simulink model "balanceCar3"  (R2023b)
settings: Solver=VariableStepAuto  StartTime=0.0  StopTime=20  RelTol=1e-3
settings Model: SimulationMode=accelerator  Creator=xjtu  LastModifiedBy=xjtu

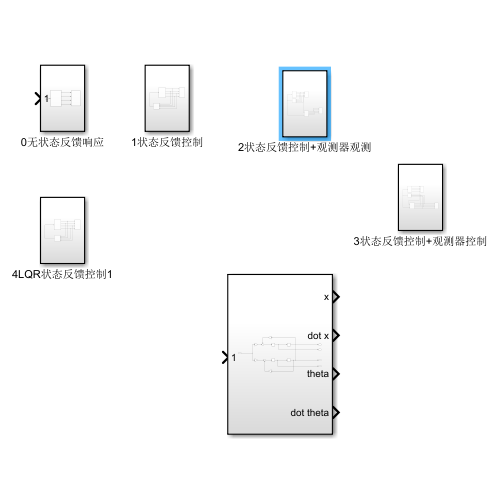
[thumbnail: Simulink's stored preview of the top-level diagram]
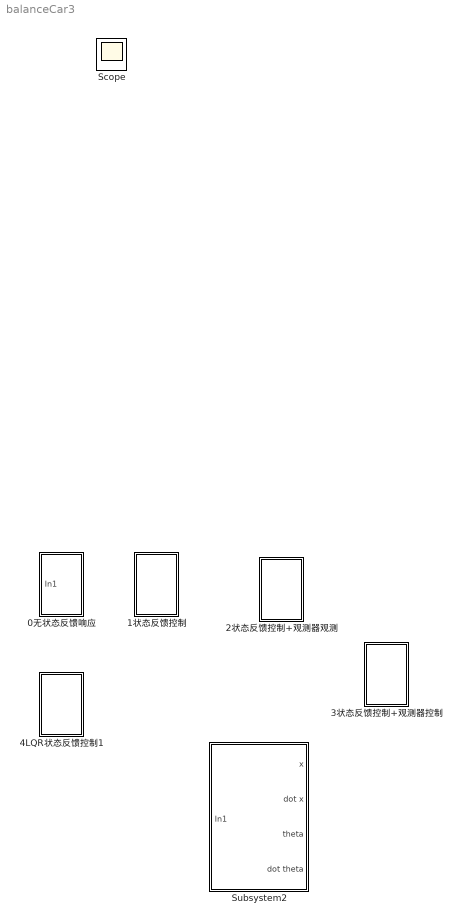
== system balanceCar3 ==
  0无状态反馈响应 : Subsystem
  1状态反馈控制 : Subsystem
  2状态反馈控制+观测器观测 : Subsystem
  3状态反馈控制+观测器控制 : Subsystem
  4LQR状态反馈控制1 : Subsystem
  Subsystem2 : Subsystem
  Scope : Scope

== system balanceCar3/0无状态反馈响应 ==
  In1 : Inport
  Scope1 : Scope  NumInputPorts=4
  Subsystem1 : Subsystem
  wires:
  Subsystem1/3(theta) -> Scope1/3
  Subsystem1/2(dot x) -> Scope1/2
  Subsystem1/4(dot theta) -> Scope1/4
  In1/1 -> Subsystem1/1(In1)
  Subsystem1/1(x) -> Scope1/1

== system balanceCar3/1状态反馈控制 ==
  1状态反馈系统模块 : Subsystem
  Scope : Scope  NumInputPorts=4
  Subsystem : Subsystem
  wires:
  Subsystem/2(dot x) -> 1状态反馈系统模块/1(dot x), Scope/2
  Subsystem/4(dot theta) -> 1状态反馈系统模块/3(dot theta), Scope/4
  1状态反馈系统模块/1(Out1) -> Subsystem/1(In1)
  Subsystem/3(theta) -> 1状态反馈系统模块/4(theta), Scope/3
  Subsystem/1(x) -> 1状态反馈系统模块/2(x), Scope/1

== system balanceCar3/2状态反馈控制+观测器观测 ==
  1状态反馈系统模块 : Subsystem
  Scope : Scope  NumInputPorts=4
  Scope1 : Scope  NumInputPorts=4
  Subsystem : Subsystem
  Subsystem1 : Subsystem
  wires:
  Subsystem/3(theta) -> Scope/3, 1状态反馈系统模块/4(theta)
  1状态反馈系统模块/1(Out1) -> Subsystem/1(In1), Subsystem1/2(u)  "u"
  Subsystem/4(dot theta) -> Scope/4, 1状态反馈系统模块/3(dot theta)
  Subsystem/2(dot x) -> Scope/2, 1状态反馈系统模块/1(dot x)
  Subsystem/1(x) -> Subsystem1/1(In1), Scope/1, 1状态反馈系统模块/2(x)
  Subsystem1/1(x hat) -> Scope1/1
  Subsystem1/2(dot x hat) -> Scope1/2
  Subsystem1/3(theta hat) -> Scope1/3
  Subsystem1/4(dot theta hat) -> Scope1/4

== system balanceCar3/3状态反馈控制+观测器控制 ==
  1状态反馈系统模块 : Subsystem
  Scope : Scope  NumInputPorts=4
  Scope1 : Scope  NumInputPorts=4
  Subsystem : Subsystem
  Subsystem1 : Subsystem
  wires:
  Subsystem1/4(dot theta hat) -> 1状态反馈系统模块/3(dot theta), Scope1/4
  Subsystem1/3(theta hat) -> 1状态反馈系统模块/4(theta), Scope1/3
  Subsystem1/2(dot x hat) -> 1状态反馈系统模块/1(dot x), Scope1/2
  Subsystem1/1(x hat) -> 1状态反馈系统模块/2(x), Scope1/1
  Subsystem/1(x) -> Scope/1, Subsystem1/1(In1)
  Subsystem/2(dot x) -> Scope/2
  Subsystem/4(dot theta) -> Scope/4
  1状态反馈系统模块/1(Out1) -> Subsystem1/2(u), Subsystem/1(In1)  "u"
  Subsystem/3(theta) -> Scope/3

== system balanceCar3/4LQR状态反馈控制1 ==
  LQR状态反馈系统模块 : Subsystem
  Scope : Scope  NumInputPorts=4
  Subsystem : Subsystem
  wires:
  Subsystem/1(x) -> Scope/1, LQR状态反馈系统模块/2(x)
  Subsystem/3(theta) -> Scope/3, LQR状态反馈系统模块/4(theta)
  LQR状态反馈系统模块/1(Out1) -> Subsystem/1(In1)
  Subsystem/4(dot theta) -> Scope/4, LQR状态反馈系统模块/3(dot theta)
  Subsystem/2(dot x) -> Scope/2, LQR状态反馈系统模块/1(dot x)

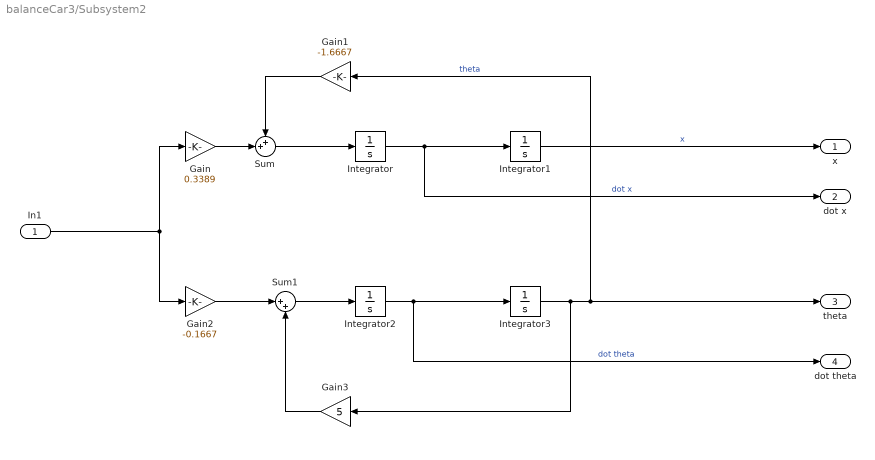
== system balanceCar3/Subsystem2 ==
  In1 : Inport
  Gain : Gain  Gain=0.3389
  Gain1 : Gain  Gain=-1.6667
  Gain2 : Gain  Gain=-0.1667
  Gain3 : Gain  Gain=5
  Integrator : Integrator
  Integrator1 : Integrator
  Integrator2 : Integrator
  Integrator3 : Integrator  InitialCondition=5/180*pi
  Sum : Sum  Inputs=++|
  Sum1 : Sum  Inputs=|++
  x : Outport
  dot x : Outport  Port=2
  theta : Outport  Port=3
  dot theta : Outport  Port=4
  wires:
  Integrator/1 -> dot x/1, Integrator1/1  "dot x"
  Gain1/1 -> Sum/1
  Sum/1 -> Integrator/1
  Integrator3/1 -> Gain3/1, Gain1/1, theta/1  "theta"
  Integrator2/1 -> dot theta/1, Integrator3/1  "dot theta"
  Gain2/1 -> Sum1/1
  Gain/1 -> Sum/2
  Sum1/1 -> Integrator2/1
  Gain3/1 -> Sum1/2
  In1/1 -> Gain/1, Gain2/1
  Integrator1/1 -> x/1  "x"

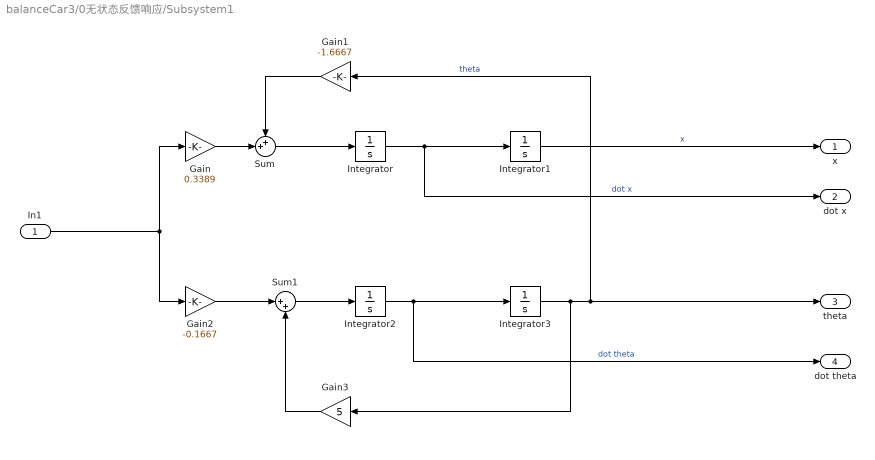
== system balanceCar3/0无状态反馈响应/Subsystem1 ==
  In1 : Inport
  Gain : Gain  Gain=0.3389
  Gain1 : Gain  Gain=-1.6667
  Gain2 : Gain  Gain=-0.1667
  Gain3 : Gain  Gain=5
  Integrator : Integrator
  Integrator1 : Integrator
  Integrator2 : Integrator
  Integrator3 : Integrator  InitialCondition=5/180*pi
  Sum : Sum  Inputs=++|
  Sum1 : Sum  Inputs=|++
  x : Outport
  dot x : Outport  Port=2
  theta : Outport  Port=3
  dot theta : Outport  Port=4
  wires:
  Integrator1/1 -> x/1  "x"
  In1/1 -> Gain2/1, Gain/1
  Gain3/1 -> Sum1/2
  Sum1/1 -> Integrator2/1
  Gain/1 -> Sum/2
  Gain2/1 -> Sum1/1
  Integrator2/1 -> Integrator3/1, dot theta/1  "dot theta"
  Integrator3/1 -> theta/1, Gain1/1, Gain3/1  "theta"
  Sum/1 -> Integrator/1
  Gain1/1 -> Sum/1
  Integrator/1 -> Integrator1/1, dot x/1  "dot x"

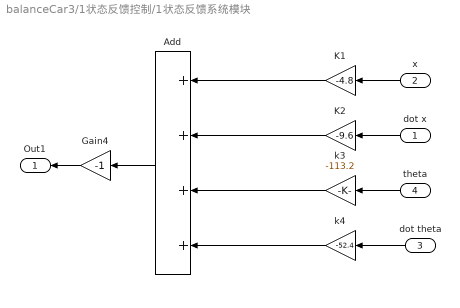
== system balanceCar3/1状态反馈控制/1状态反馈系统模块 ==
  dot x : Inport
  x : Inport  Port=2
  dot theta : Inport  Port=3
  theta : Inport  Port=4
  Add : Sum  Inputs=++++
  Gain4 : Gain  Gain=-1
  K1 : Gain  Gain=-4.8
  K2 : Gain  Gain=-9.6
  k3 : Gain  Gain=-113.2
  k4 : Gain  Gain=-52.4
  Out1 : Outport
  wires:
  k3/1 -> Add/3
  dot theta/1 -> k4/1
  Add/1 -> Gain4/1
  K1/1 -> Add/1
  theta/1 -> k3/1
  k4/1 -> Add/4
  x/1 -> K1/1
  dot x/1 -> K2/1
  K2/1 -> Add/2
  Gain4/1 -> Out1/1

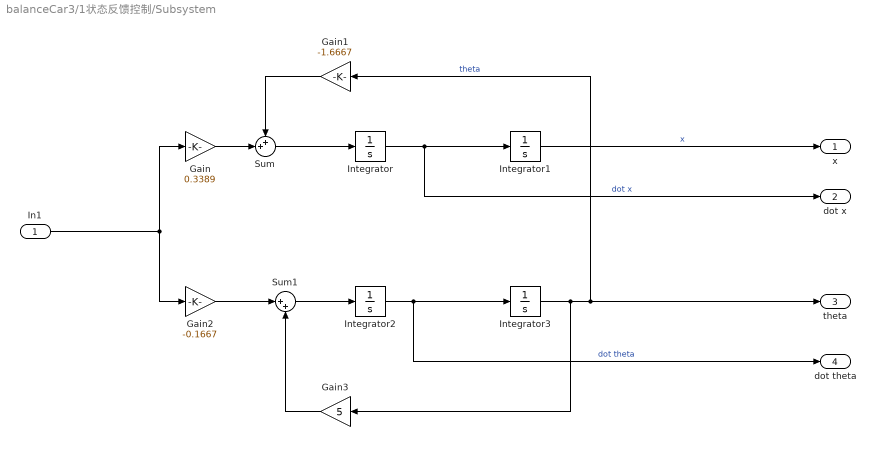
== system balanceCar3/1状态反馈控制/Subsystem ==
  In1 : Inport
  Gain : Gain  Gain=0.3389
  Gain1 : Gain  Gain=-1.6667
  Gain2 : Gain  Gain=-0.1667
  Gain3 : Gain  Gain=5
  Integrator : Integrator
  Integrator1 : Integrator
  Integrator2 : Integrator
  Integrator3 : Integrator  InitialCondition=5/180*pi
  Sum : Sum  Inputs=++|
  Sum1 : Sum  Inputs=|++
  x : Outport
  dot x : Outport  Port=2
  theta : Outport  Port=3
  dot theta : Outport  Port=4
  wires:
  Integrator/1 -> dot x/1, Integrator1/1  "dot x"
  Gain1/1 -> Sum/1
  Sum/1 -> Integrator/1
  Integrator3/1 -> Gain3/1, Gain1/1, theta/1  "theta"
  Integrator2/1 -> dot theta/1, Integrator3/1  "dot theta"
  Gain2/1 -> Sum1/1
  Gain/1 -> Sum/2
  Sum1/1 -> Integrator2/1
  Gain3/1 -> Sum1/2
  In1/1 -> Gain/1, Gain2/1
  Integrator1/1 -> x/1  "x"

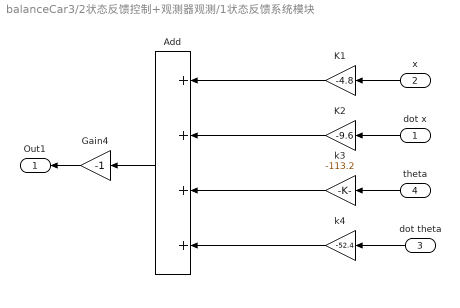
== system balanceCar3/2状态反馈控制+观测器观测/1状态反馈系统模块 ==
  dot x : Inport
  x : Inport  Port=2
  dot theta : Inport  Port=3
  theta : Inport  Port=4
  Add : Sum  Inputs=++++
  Gain4 : Gain  Gain=-1
  K1 : Gain  Gain=-4.8
  K2 : Gain  Gain=-9.6
  k3 : Gain  Gain=-113.2
  k4 : Gain  Gain=-52.4
  Out1 : Outport
  wires:
  Gain4/1 -> Out1/1
  K2/1 -> Add/2
  dot x/1 -> K2/1
  x/1 -> K1/1
  k4/1 -> Add/4
  theta/1 -> k3/1
  K1/1 -> Add/1
  Add/1 -> Gain4/1
  dot theta/1 -> k4/1
  k3/1 -> Add/3

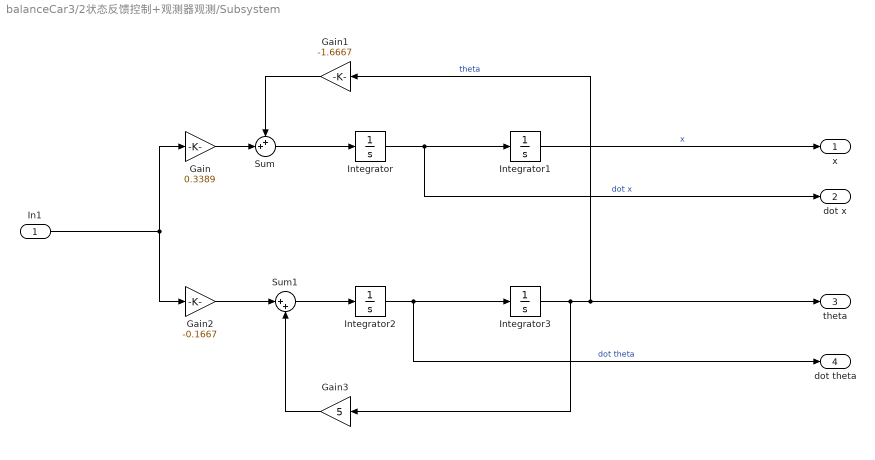
== system balanceCar3/2状态反馈控制+观测器观测/Subsystem ==
  In1 : Inport
  Gain : Gain  Gain=0.3389
  Gain1 : Gain  Gain=-1.6667
  Gain2 : Gain  Gain=-0.1667
  Gain3 : Gain  Gain=5
  Integrator : Integrator
  Integrator1 : Integrator
  Integrator2 : Integrator
  Integrator3 : Integrator  InitialCondition=5/180*pi
  Sum : Sum  Inputs=++|
  Sum1 : Sum  Inputs=|++
  x : Outport
  dot x : Outport  Port=2
  theta : Outport  Port=3
  dot theta : Outport  Port=4
  wires:
  Integrator1/1 -> x/1  "x"
  In1/1 -> Gain2/1, Gain/1
  Gain3/1 -> Sum1/2
  Sum1/1 -> Integrator2/1
  Gain/1 -> Sum/2
  Gain2/1 -> Sum1/1
  Integrator2/1 -> Integrator3/1, dot theta/1  "dot theta"
  Integrator3/1 -> theta/1, Gain1/1, Gain3/1  "theta"
  Sum/1 -> Integrator/1
  Gain1/1 -> Sum/1
  Integrator/1 -> Integrator1/1, dot x/1  "dot x"

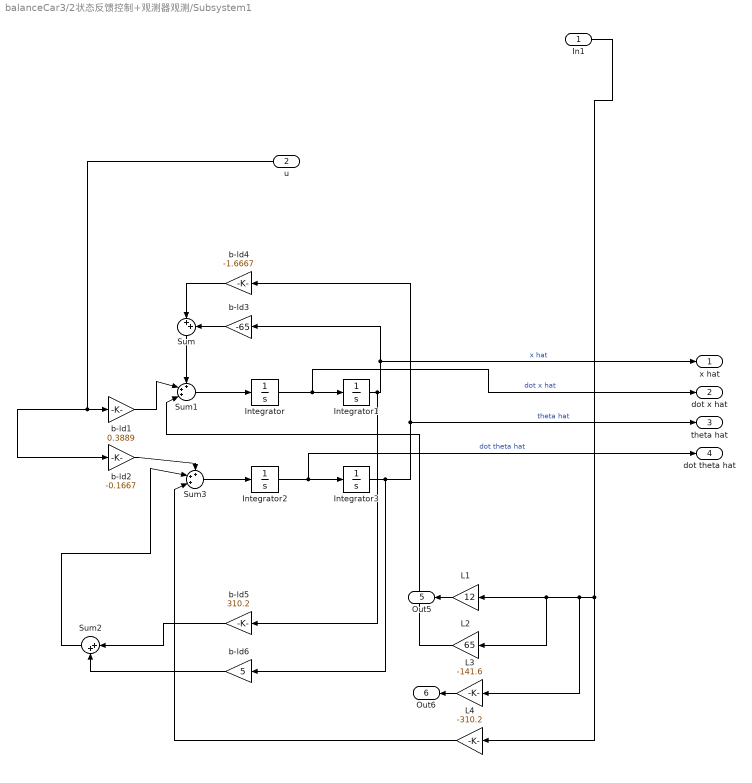
== system balanceCar3/2状态反馈控制+观测器观测/Subsystem1 ==
  In1 : Inport
  u : Inport  Port=2
  Integrator : Integrator
  Integrator1 : Integrator
  Integrator2 : Integrator
  Integrator3 : Integrator  InitialCondition=5/180*pi
  L1 : Gain  Gain=12
  L2 : Gain  Gain=65
  L3 : Gain  Gain=-141.6
  L4 : Gain  Gain=-310.2
  Sum : Sum  Inputs=|++
  Sum1 : Sum  Inputs=+++|
  Sum2 : Sum  Inputs=|++
  Sum3 : Sum  Inputs=+++|
  b-ld1 : Gain  Gain=0.3889
  b-ld2 : Gain  Gain=-0.1667
  b-ld3 : Gain  Gain=-65
  b-ld4 : Gain  Gain=-1.6667
  b-ld5 : Gain  Gain=310.2
  b-ld6 : Gain  Gain=5
  x hat : Outport
  dot x hat : Outport  Port=2
  theta hat : Outport  Port=3
  dot theta hat : Outport  Port=4
  Out5 : Outport  Port=5
  Out6 : Outport  Port=6
  wires:
  Integrator1/1 -> x hat/1, b-ld3/1, b-ld5/1  "x hat"
  b-ld6/1 -> Sum2/2
  Integrator2/1 -> dot theta hat/1, Integrator3/1  "dot theta hat"
  Integrator3/1 -> b-ld6/1, theta hat/1, b-ld4/1  "theta hat"
  b-ld2/1 -> Sum3/1
  In1/1 -> L4/1, L3/1, L2/1, L1/1
  b-ld4/1 -> Sum/1
  b-ld1/1 -> Sum1/2
  L2/1 -> Sum1/3
  b-ld3/1 -> Sum/2
  Integrator/1 -> dot x hat/1, Integrator1/1  "dot x hat"
  L3/1 -> Out6/1
  Sum2/1 -> Sum3/2
  L4/1 -> Sum3/3
  L1/1 -> Out5/1
  b-ld5/1 -> Sum2/1
  Sum/1 -> Sum1/1
  Sum1/1 -> Integrator/1
  Sum3/1 -> Integrator2/1
  u/1 -> b-ld2/1, b-ld1/1

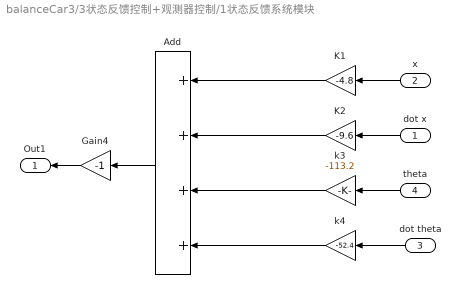
== system balanceCar3/3状态反馈控制+观测器控制/1状态反馈系统模块 ==
  dot x : Inport
  x : Inport  Port=2
  dot theta : Inport  Port=3
  theta : Inport  Port=4
  Add : Sum  Inputs=++++
  Gain4 : Gain  Gain=-1
  K1 : Gain  Gain=-4.8
  K2 : Gain  Gain=-9.6
  k3 : Gain  Gain=-113.2
  k4 : Gain  Gain=-52.4
  Out1 : Outport
  wires:
  k3/1 -> Add/3
  dot theta/1 -> k4/1
  Add/1 -> Gain4/1
  K1/1 -> Add/1
  theta/1 -> k3/1
  k4/1 -> Add/4
  x/1 -> K1/1
  dot x/1 -> K2/1
  K2/1 -> Add/2
  Gain4/1 -> Out1/1

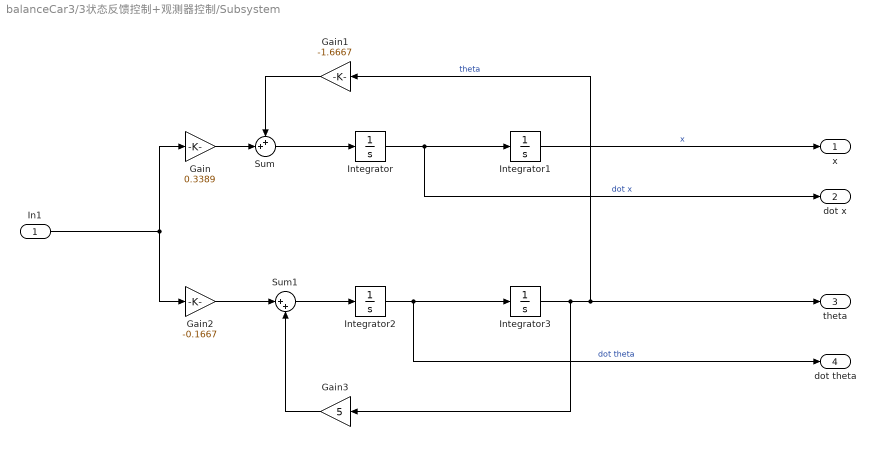
== system balanceCar3/3状态反馈控制+观测器控制/Subsystem ==
  In1 : Inport
  Gain : Gain  Gain=0.3389
  Gain1 : Gain  Gain=-1.6667
  Gain2 : Gain  Gain=-0.1667
  Gain3 : Gain  Gain=5
  Integrator : Integrator
  Integrator1 : Integrator
  Integrator2 : Integrator
  Integrator3 : Integrator  InitialCondition=5/180*pi
  Sum : Sum  Inputs=++|
  Sum1 : Sum  Inputs=|++
  x : Outport
  dot x : Outport  Port=2
  theta : Outport  Port=3
  dot theta : Outport  Port=4
  wires:
  Integrator/1 -> dot x/1, Integrator1/1  "dot x"
  Gain1/1 -> Sum/1
  Sum/1 -> Integrator/1
  Integrator3/1 -> Gain3/1, Gain1/1, theta/1  "theta"
  Integrator2/1 -> dot theta/1, Integrator3/1  "dot theta"
  Gain2/1 -> Sum1/1
  Gain/1 -> Sum/2
  Sum1/1 -> Integrator2/1
  Gain3/1 -> Sum1/2
  In1/1 -> Gain/1, Gain2/1
  Integrator1/1 -> x/1  "x"

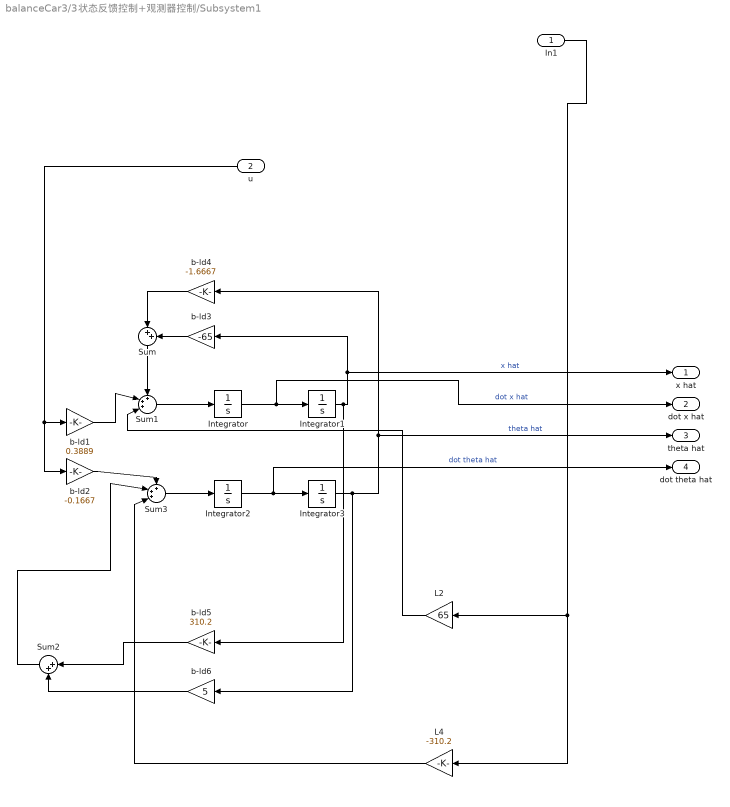
== system balanceCar3/3状态反馈控制+观测器控制/Subsystem1 ==
  In1 : Inport
  u : Inport  Port=2
  Integrator{,1..3} (4 alike) : Integrator
  L2 : Gain  Gain=65
  L4 : Gain  Gain=-310.2
  Sum : Sum  Inputs=|++
  Sum1 : Sum  Inputs=+++|
  Sum2 : Sum  Inputs=|++
  Sum3 : Sum  Inputs=+++|
  b-ld1 : Gain  Gain=0.3889
  b-ld2 : Gain  Gain=-0.1667
  b-ld3 : Gain  Gain=-65
  b-ld4 : Gain  Gain=-1.6667
  b-ld5 : Gain  Gain=310.2
  b-ld6 : Gain  Gain=5
  x hat : Outport
  dot x hat : Outport  Port=2
  theta hat : Outport  Port=3
  dot theta hat : Outport  Port=4
  wires:
  u/1 -> b-ld1/1, b-ld2/1
  Sum3/1 -> Integrator2/1
  Sum1/1 -> Integrator/1
  Sum/1 -> Sum1/1
  b-ld5/1 -> Sum2/1
  L4/1 -> Sum3/3
  Sum2/1 -> Sum3/2
  Integrator/1 -> Integrator1/1, dot x hat/1  "dot x hat"
  b-ld3/1 -> Sum/2
  L2/1 -> Sum1/3
  b-ld1/1 -> Sum1/2
  b-ld4/1 -> Sum/1
  In1/1 -> L2/1, L4/1
  b-ld2/1 -> Sum3/1
  Integrator3/1 -> b-ld4/1, theta hat/1, b-ld6/1  "theta hat"
  Integrator2/1 -> Integrator3/1, dot theta hat/1  "dot theta hat"
  b-ld6/1 -> Sum2/2
  Integrator1/1 -> b-ld5/1, b-ld3/1, x hat/1  "x hat"

== system balanceCar3/4LQR状态反馈控制1/LQR状态反馈系统模块 ==
  dot x : Inport
  x : Inport  Port=2
  dot theta : Inport  Port=3
  theta : Inport  Port=4
  Add : Sum  Inputs=++++
  Gain4 : Gain  Gain=-1
  K1 : Gain  Gain=-1
  K2 : Gain  Gain=-3.5558
  k3 : Gain  Gain=-88.2203
  k4 : Gain  Gain=-40.5008
  Out1 : Outport
  wires:
  Gain4/1 -> Out1/1
  K2/1 -> Add/2
  dot x/1 -> K2/1
  x/1 -> K1/1
  k4/1 -> Add/4
  theta/1 -> k3/1
  K1/1 -> Add/1
  Add/1 -> Gain4/1
  dot theta/1 -> k4/1
  k3/1 -> Add/3

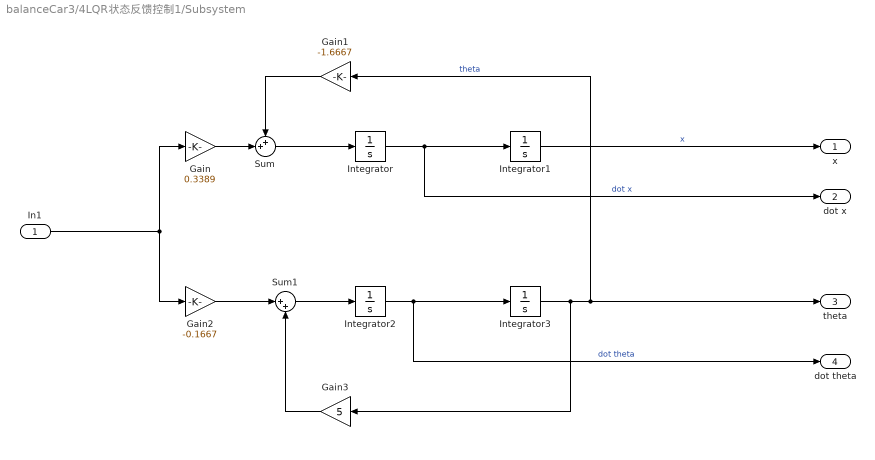
== system balanceCar3/4LQR状态反馈控制1/Subsystem ==
  In1 : Inport
  Gain : Gain  Gain=0.3389
  Gain1 : Gain  Gain=-1.6667
  Gain2 : Gain  Gain=-0.1667
  Gain3 : Gain  Gain=5
  Integrator : Integrator
  Integrator1 : Integrator
  Integrator2 : Integrator
  Integrator3 : Integrator  InitialCondition=5/180*pi
  Sum : Sum  Inputs=++|
  Sum1 : Sum  Inputs=|++
  x : Outport
  dot x : Outport  Port=2
  theta : Outport  Port=3
  dot theta : Outport  Port=4
  wires:
  Integrator1/1 -> x/1  "x"
  In1/1 -> Gain2/1, Gain/1
  Gain3/1 -> Sum1/2
  Sum1/1 -> Integrator2/1
  Gain/1 -> Sum/2
  Gain2/1 -> Sum1/1
  Integrator2/1 -> Integrator3/1, dot theta/1  "dot theta"
  Integrator3/1 -> theta/1, Gain1/1, Gain3/1  "theta"
  Sum/1 -> Integrator/1
  Gain1/1 -> Sum/1
  Integrator/1 -> Integrator1/1, dot x/1  "dot x"
